simulink model "History1_tmp"  (Simulink 8.3)
settings: Solver=ode45  StartTime=0.0  StopTime=10.0  RelTol=1e-3
settings Model: Creator=scaife  LastModifiedBy=hbourbou  CovSFcnEnable=on  ExtModeAutoUpdateStatusClock=off
settings DataIOCC: SignalLoggingName=sigsOut
settings DebuggingCC: SaveWithParameterizedLinksMsg=none  SignalResolutionControl=TryResolveAllWithWarning  SolverPrmCheckMsg=none  MultiTaskDSMMsg=warning  MultiTaskCondExecSysMsg=none  FrameProcessingCompatibilityMsg=error  StateNameClashWarn=none  SFUnexpectedBacktrackingDiag=error  SFNoUnconditionalDefaultTransitionDiag=error
settings HardwareCC: TargetUnknown=on
settings SFSimCC: SimParseCustomCode=off
settings GRTTargetCC: GeneratePreprocessorConditionals=Use local settings

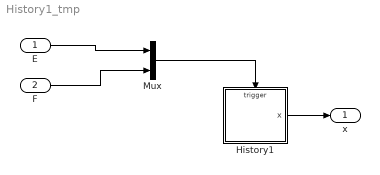
== system History1_tmp ==
  E : Inport
  F : Inport  Port=2
  History1 : Stateflow chart  TreatAsAtomicUnit=on
      settings: PermitHierarchicalResolution=ParametersOnly
  Mux : Mux  Inputs=2
  x : Outport
  wires:
  E/1 -> Mux/1
  F/1 -> Mux/2
  Mux/1 -> History1/Trigger
  History1/1(x) -> x/1

== stateflow chart History1 ==
  state A
    (history)
    state A1/
      en: x+=1;
      ex: x-=1;
    state A2/
      en: x+=10;
      ex: x-=10;
    (default) -> A1
    A2 -> A1 : E
    A1 -> A2 : E
  state B
    (history)
    state B1/
      en: x+=100;
      ex: x-=100;
    state B2/
      en: x+=1000;
      ex: x-=1000;
    (default) -> B1
    B2 -> B1 : E
    B1 -> B2 : E
  (default) -> A
  A -> B : F
  B -> A : F
  data: x output int32
  events: E input EITHER_EDGE_EVENT; F input EITHER_EDGE_EVENT
